simulink model "ammclib_gflib_trigonometric_s32k11x"  (Simulink 9.0)
settings: Solver=FixedStepDiscrete  StartTime=0.0  StopTime=5  FixedStep=0.001  RelTol=1e-3  EnableMultiTasking=on
InitFcn:
  | mbd_s32k_consistency_checks(bdroot(gcs));
undefined symbols (not defined in the file): LQFP, thumb
libraries: ammclib_bam_s32k11x x23, mbd_s32k1xx_ec_toolbox x2, simulink x1
Description:
  | This model tests the AMMCLIB GFLIB TRIGONOMETRIC blocks
  | 
  | Validation:
  | - Run the model in Simulation and check the results
  | - Open Freemaster (ammclib_gflib_trigonometric_s32k11x.pmp) and compare the HW results against the Simulated ones
CloseFcn:
  | clear all;
settings Model: Creator=NXP MBDT Team  LastModifiedBy=nxf35172
settings DataIOCC: ExternalInput=off  InitialState=off  LimitDataPoints=on  SaveOutput=off  SignalLogging=off  SaveTime=off
settings OptimizationCC: DefaultParameterBehavior=Inlined  PassReuseOutputArgsAs=Individual arguments  LifeSpan=auto
settings DebuggingCC: SolverPrmCheckMsg=warning  InheritedTsInSrcMsg=none  SingleTaskRateTransMsg=error  IntegerOverflowMsg=none  ParameterPrecisionLossMsg=none  ParameterTunabilityLossMsg=error  UnconnectedInputMsg=error  UnconnectedOutputMsg=error  UnconnectedLineMsg=error  AllowSymbolicDim=off  UnknownTsInhSupMsg=error  StateNameClashWarn=warning
settings HardwareCC: ProdLargestAtomicInteger=Long  ProdLargestAtomicFloat=Double  ProdIntDivRoundTo=Zero  ProdEndianess=LittleEndian  ProdHWDeviceType=ARM Compatible->ARM Cortex
settings SFSimCC: MATLABDynamicMemAlloc=off
settings RTWCC: SystemTargetFile=mbd_s32k.tlc  MakeCommand=mbd_s32k_make_rtw COPY_MDLREF_INCLUDES=0  TemplateMakefile=mbd_s32k.tmf  Description=Model Based Design Toolbox S32K14x Code Generation Target  GenerateReport=on  IncludeHyperlinkInReport=on  LaunchReport=on  GenerateTraceInfo=on  GenerateTraceReport=on  GenerateTraceReportSl=on  GenerateTraceReportSf=on  GenerateTraceReportEml=on
settings CodeAppCC: ForceParamTrailComments=on  IgnoreCustomStorageClasses=off  OperatorAnnotations=on  SimulinkDataObjDesc=on  SFDataObjDesc=on  InsertBlockDesc=on  StateflowObjectComments=off
settings STFCustomTargetCC: MultiwordLength=256  ModelReferenceCompliant=off  CombineOutputUpdateFcns=on  ERTCustomFileBanners=on  SupportContinuousTime=off  SupportNonInlinedSFcns=off  RemoveResetFunc=on  MATLABClassNameForMDSCustomization=Simulink.SoftwareTarget.ERTCustomization  GRTInterface=off  SystemTargetFile=mbd_s32k.tlc
settings ERTTargetCC: ModelReferenceCompliant=off  ParMdlRefBuildCompliant=off  CompOptLevelCompliant=off  ConcurrentExecutionCompliant=off  ModelStepFunctionPrototypeControlCompliant=off  CPPClassGenCompliant=off  UseToolchainInfoCompliant=off  InlinedParameterPlacement=NonHierarchical  ERTCustomFileTemplate=example_file_process.tlc

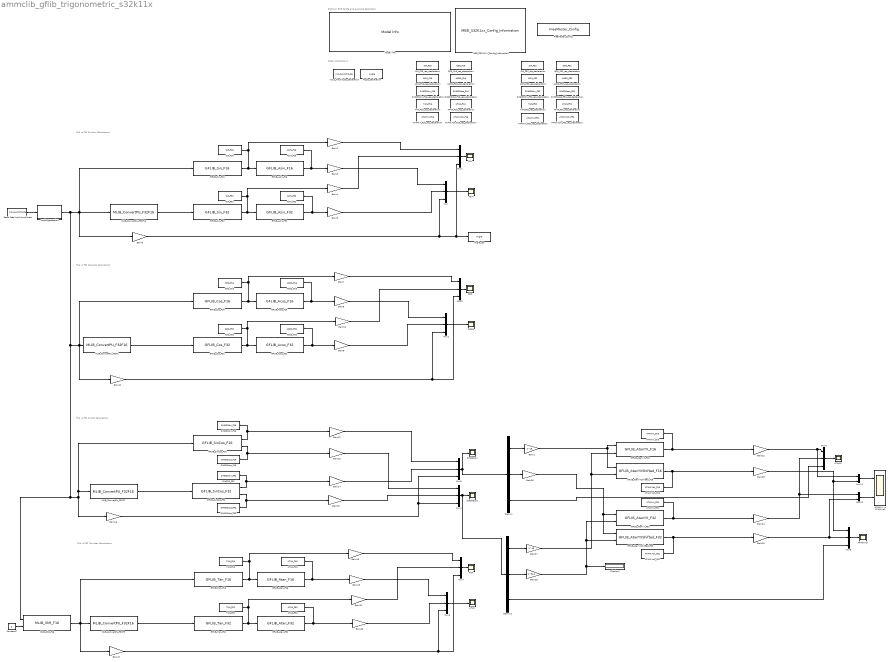
== system ammclib_gflib_trigonometric_s32k11x ==
  note: S32K11x EVB Config and example description
  note: Data Initializations
  note: F16 vs F32 Sin/Asin Calculations
  note: F16 vs F32 Cos/Acos Calculations
  note: F16 vs F32 SinCos Calculations
  note: F16 vs F32 Tan/Atan Calculations
  ACOS : Scope
  ACOS_F16 : DataStoreWrite  DataStoreName=ACOS_F16
  ACOS_F16_res_declaration : DataStoreMemory  Priority=2  DataStoreName=ACOS_F16  ReadBeforeWriteMsg=warning  WriteAfterWriteMsg=warning  WriteAfterReadMsg=warning  ShowAdditionalParam=off  OutDataTypeStr=int16
  ACOS_F32 : DataStoreWrite  DataStoreName=ACOS_F32
  ACOS_F32_res_declaration : DataStoreMemory  Priority=2  DataStoreName=ACOS_F32  ReadBeforeWriteMsg=warning  WriteAfterWriteMsg=warning  WriteAfterReadMsg=warning  ShowAdditionalParam=off  OutDataTypeStr=int32
  ASIN : Scope
  ASIN_F16 : DataStoreWrite  DataStoreName=ASIN_F16
  ASIN_F16_res_declaration : DataStoreMemory  Priority=2  DataStoreName=ASIN_F16  ReadBeforeWriteMsg=warning  WriteAfterWriteMsg=warning  WriteAfterReadMsg=warning  ShowAdditionalParam=off  OutDataTypeStr=int16
  ASIN_F32 : DataStoreWrite  DataStoreName=ASIN_F32
  ASIN_F32_res_declaration : DataStoreMemory  Priority=2  DataStoreName=ASIN_F32  ReadBeforeWriteMsg=warning  WriteAfterWriteMsg=warning  WriteAfterReadMsg=warning  ShowAdditionalParam=off  OutDataTypeStr=int32
  ATAN : Scope
  ATANXY : Scope
  ATANXYsh : Scope
  ATANYX vs ATANXYsh : Scope  NumInputPorts=2
  ATANYX_F16 : DataStoreWrite  DataStoreName=ATANYX_F16
  ATANYX_F16_res_declaration : DataStoreMemory  Priority=2  DataStoreName=ATANYX_F16  ReadBeforeWriteMsg=warning  WriteAfterWriteMsg=warning  WriteAfterReadMsg=warning  ShowAdditionalParam=off  OutDataTypeStr=int16
  ATANYX_F32 : DataStoreWrite  DataStoreName=ATANYX_F32
  ATANYX_F32_res_declaration : DataStoreMemory  Priority=2  DataStoreName=ATANYX_F32  ReadBeforeWriteMsg=warning  WriteAfterWriteMsg=warning  WriteAfterReadMsg=warning  ShowAdditionalParam=off  OutDataTypeStr=int32
  ATANYXsh_F16 : DataStoreWrite  DataStoreName=ATANYXsh_F16
  ATANYXsh_F16_res_declaration : DataStoreMemory  Priority=2  DataStoreName=ATANYXsh_F16  ReadBeforeWriteMsg=warning  WriteAfterWriteMsg=warning  WriteAfterReadMsg=warning  ShowAdditionalParam=off  OutDataTypeStr=int16
  ATANYXsh_F32 : DataStoreWrite  DataStoreName=ATANYXsh_F32
  ATANYXsh_F32_res_declaration : DataStoreMemory  Priority=2  DataStoreName=ATANYXsh_F32  ReadBeforeWriteMsg=warning  WriteAfterWriteMsg=warning  WriteAfterReadMsg=warning  ShowAdditionalParam=off  OutDataTypeStr=int32
  ATAN_F16 : DataStoreWrite  DataStoreName=ATAN_F16
  ATAN_F16_res_declaration : DataStoreMemory  Priority=2  DataStoreName=ATAN_F16  ReadBeforeWriteMsg=warning  WriteAfterWriteMsg=warning  WriteAfterReadMsg=warning  ShowAdditionalParam=off  OutDataTypeStr=int16
  ATAN_F32 : DataStoreWrite  DataStoreName=ATAN_F32
  ATAN_F32_res_declaration : DataStoreMemory  Priority=2  DataStoreName=ATAN_F32  ReadBeforeWriteMsg=warning  WriteAfterWriteMsg=warning  WriteAfterReadMsg=warning  ShowAdditionalParam=off  OutDataTypeStr=int32
  Angle generation : Subsystem
  Angle_declaration : DataStoreMemory  Priority=1  DataStoreName=Angle  WriteAfterWriteMsg=warning  WriteAfterReadMsg=warning  ShowAdditionalParam=off  OutMin=-1  OutMax=1  OutDataTypeStr=single
  Angle_res : DataStoreWrite  DataStoreName=Angle
  COS : Scope
  COS_F16 : DataStoreWrite  DataStoreName=COS_F16
  COS_F16_res_declaration : DataStoreMemory  Priority=2  DataStoreName=COS_F16  ReadBeforeWriteMsg=warning  WriteAfterWriteMsg=warning  WriteAfterReadMsg=warning  ShowAdditionalParam=off  OutDataTypeStr=int16
  COS_F32 : DataStoreWrite  DataStoreName=COS_F32
  COS_F32_res_declaration : DataStoreMemory  Priority=2  DataStoreName=COS_F32  ReadBeforeWriteMsg=warning  WriteAfterWriteMsg=warning  WriteAfterReadMsg=warning  ShowAdditionalParam=off  OutDataTypeStr=int32
  Constant7 : Constant  Value=2  OutDataTypeStr=Inherit: Inherit via back propagation
  Demux : Demux  Outputs=3
  Demux1 : Demux  Outputs=3
  Display2 : Display
  FreeMaster_Config : mbd_s32k1xx_ec_toolbox/Utility Blocks/FreeMaster_Config  interface=LPUART0  baudrate=19200  rxd=PTB0: [LPUART0_RX | Receive]  txd=PTB1: [LPUART0_TX | Transmit]  mode=Short Interrupt  isr_prio=3  show_adv_opts=on  use_scope=on  max_scope_vars=8  use_recorder=on  max_rec_vars=8  rec_buff_size=1024  rec_timebase=0 seconds  comm_buffer_size_auto=on  comm_buffer_size=255  comm_rqueue_size_default=on  comm_rqueue_size=32
  GFLIB_Acos_F16 : ammclib_bam_s32k11x/GFLIB/bam_f16/GFLIB_Acos_F16
  GFLIB_Acos_F32 : ammclib_bam_s32k11x/GFLIB/bam_f32/GFLIB_Acos_F32
  GFLIB_Asin_F16 : ammclib_bam_s32k11x/GFLIB/bam_f16/GFLIB_Asin_F16
  GFLIB_Asin_F32 : ammclib_bam_s32k11x/GFLIB/bam_f32/GFLIB_Asin_F32
  GFLIB_AtanYXShifted_F16 : ammclib_bam_s32k11x/GFLIB/bam_f16/GFLIB_AtanYXShifted_F16  Ky=19918  Kx=28803  Ny=0  Nx=0  ThetaAdj=1820
  GFLIB_AtanYXShifted_F32 : ammclib_bam_s32k11x/GFLIB/bam_f32/GFLIB_AtanYXShifted_F32  Ky=1.305434611595101e+09  Kx=1.887749824036660e+09  Ny=0  Nx=0  ThetaAdj=1.193046470436251e+08
  GFLIB_AtanYX_F16 : ammclib_bam_s32k11x/GFLIB/bam_f16/GFLIB_AtanYX_F16
  GFLIB_AtanYX_F32 : ammclib_bam_s32k11x/GFLIB/bam_f32/GFLIB_AtanYX_F32
  GFLIB_Atan_F16 : ammclib_bam_s32k11x/GFLIB/bam_f16/GFLIB_Atan_F16
  GFLIB_Atan_F32 : ammclib_bam_s32k11x/GFLIB/bam_f32/GFLIB_Atan_F32
  GFLIB_Cos_F16 : ammclib_bam_s32k11x/GFLIB/bam_f16/GFLIB_Cos_F16
  GFLIB_Cos_F32 : ammclib_bam_s32k11x/GFLIB/bam_f32/GFLIB_Cos_F32
  GFLIB_SinCos_F16 : ammclib_bam_s32k11x/GFLIB/bam_f16/GFLIB_SinCos_F16
  GFLIB_SinCos_F32 : ammclib_bam_s32k11x/GFLIB/bam_f32/GFLIB_SinCos_F32
  GFLIB_Sin_F16 : ammclib_bam_s32k11x/GFLIB/bam_f16/GFLIB_Sin_F16
  GFLIB_Sin_F32 : ammclib_bam_s32k11x/GFLIB/bam_f32/GFLIB_Sin_F32
  GFLIB_Tan_F16 : ammclib_bam_s32k11x/GFLIB/bam_f16/GFLIB_Tan_F16
  GFLIB_Tan_F32 : ammclib_bam_s32k11x/GFLIB/bam_f32/GFLIB_Tan_F32
  Gain1 : Gain  Gain=2^15  OutDataTypeStr=int16
  Gain10 : Gain  Gain=1/(2^31)  OutDataTypeStr=single
  Gain{3,6,8,11,16..17,19} (7 alike) : Gain  Gain=pi/(2^15)  OutDataTypeStr=single
  Gain{2,7,12..13,18,22..23} (7 alike) : Gain  Gain=1/(2^15)  OutDataTypeStr=single
  Gain14 : Gain  Gain=1/(2^31-1)  ParamDataTypeStr=double  OutDataTypeStr=single
  Gain15 : Gain  Gain=1/(2^31-1)  ParamDataTypeStr=double  OutDataTypeStr=single
  Gain20 : Gain  Gain=pi/(2^31)  OutDataTypeStr=single
  Gain21 : Gain  Gain=1/(2^31)  OutDataTypeStr=single
  Gain24 : Gain  Gain=1/(2^31)  ParamDataTypeStr=double  OutDataTypeStr=single
  Gain25 : Gain  Gain=1/(2^31-1)  ParamDataTypeStr=double  OutDataTypeStr=single
  Gain26 : Gain  Gain=(2^31-1)  ParamDataTypeStr=double  OutDataTypeStr=int32
  Gain27 : Gain  Gain=2^15  ParamDataTypeStr=int32  OutDataTypeStr=int16
  Gain28 : Gain  Gain=2^31-1  ParamDataTypeStr=double  OutDataTypeStr=int32
  Gain4 : Gain  Gain=1/(2^31)  OutDataTypeStr=single
  Gain5 : Gain  Gain=pi/(2^31)  OutDataTypeStr=single
  Gain9 : Gain  Gain=pi/(2^31)  OutDataTypeStr=single
  Input_Amplitude_declaration : DataStoreMemory  Priority=1  DataStoreName=Input_Amplitude  WriteAfterWriteMsg=warning  WriteAfterReadMsg=warning  InitialValue=3.14  ShowAdditionalParam=off  OutMin=-pi  OutMax=pi  OutDataTypeStr=single
  MBD_S32K11x_Config_Information : mbd_s32k1xx_ec_toolbox/MBD_S32K1xx_Config_Information  mbdt_ver=0  disp_str=|  config_params=[]  mcu_target_name=S32K116  mcu_target_package=48-LQFP  mcu_target_sram_size=17KB  mcu_system_clock_freq=40  mcu_xtal_freq=External 40  mcu_steptick_timer=LPIT Channel 0  mcu_steptick_prio=3  ds_import_enable=on  target_compiler=GCC  target_memory=FLASH  gcc_target_compile_opts=-mcpu=cortex-m0plus -mthumb -O1 -g -gstrict-dwarf  gcc_target_assemble_opts=-mcpu=cortex-m0plus -mthumb -g  gcc_target_link_opts=-mcpu=cortex-m0plus -mthumb  gcc_target_default_lcf=on  gcc_target_user_lcf=S32K116_17_flash.ld  ghs_target_compile_opts=-mcpu=cortexm0plus -mthumb -fsoft -Ogeneral -Wundef -Wimplicit-int -Wshadow -Wtrigraphs --no_commons --gnu_asm -gnu99 -gdwarf-2 -G  ghs_target_assemble_opts=-mcpu=cortexm0plus -mthumb -fsoft --gnu_asm  ghs_target_link_opts=-mcpu=cortexm0plus -mthumb -fsoft  ghs_target_default_lcf=on  ghs_target_user_lcf=S32K116_17_flash.ld  iar_target_compile_opts=--thumb -Ol -e --debug --dlib_config normal  iar_target_assemble_opts=--thumb  iar_target_link_opts=--no_exceptions --vfe --inline  iar_target_default_lcf=on  iar_target_user_lcf=S32K116_17_flash.icf  pil_download_enable=off  rbl_download_enable=on  rbl_start_delay=5000  rbl_download_interface=OpenSDA  rbl_restart_request=off  rbl_com_port=Custom  rbl_com_port_custom=COM1  pil_download_rate=57600  pil_opensda_drive=Custom  pil_opensda_drive_custom=D  pil_uart_instance=0  pil_uart_rx=PTB0: [LPUART0_RX | Receive]  pil_uart_tx=PTB1: [LPUART0_TX | Transmit]  FTM_PWM_PcrCheckEnDis=on  FTM_Input_Edge_Inputs_PcrCheckEnDis=on  FTM_Dual_Edge_Inputs_PcrCheckEnDis=on  FTM_Quadrature_Inputs_PcrCheckEnDis=on  FTM_Hall_Sensor_Inputs_PcrCheckEnDis=on  LPTMR_PcrCheckEnDis=on  PIT_PcrCheckEnDis=on  RTC_PcrCheckEnDis=on  FlexCAN_PcrCheckEnDis=on  LIN_PcrCheckEnDis=on  FlexIO_PcrCheckEnDis=on  LPI2C_PcrCheckEnDis=on  LPSPI_PcrCheckEnDis=on  LPUART_PcrCheckEnDis=on  CMP_PcrCheckEnDis=on  GPIO_OutputPcrCheckEnDis=on  GPIO_InputPcrCheckEnDis=on  SBC_PcrCheckEnDis=on  AMMCLIB_PcrCheckEnDis=on  FM_PcrCheckEnDis=on  Profile_PcrCheckEnDis=on  ConfigParams_PcrCheckEnDis=on  ModelRef_PcrCheckEnDis=on  PDB0_PcrCheckEnDis=on  CSEc_PcrCheckEnDis=on  eDMA_PcrCheckEnDis=on  ADC_PcrCheckEnDis=on  WDOG_PcrCheckEnDis=on
      | Target : S32K144-64KB_SRAM
      | Package : 100-pin
      | System clock : 80 MHz
      | XTAL clock : External 8 MHz
      | Compiler : IAR
      | Target Type : FLASH
      | Download Code after build : off
      | Step Tick Interrupt Priority : 15
  MLIB_ConvertPU_F32F{1..3,16} (4 alike) : ammclib_bam_s32k11x/MLIB/bam_f32/MLIB_ConvertPU_F32F16
  MLIB_ShR_F16 : ammclib_bam_s32k11x/MLIB/bam_f16/MLIB_ShR_F16
  Model Info : simulink/Model-Wide Utilities/Model Info  Frame=off  DisplayStringWithTags=|  HorizontalTextAlignment=Left  LeftAlignmentValue=0.02
      | Model Name: %<ModelName>
      | 
      | Description: %<Description>
  Mux{,1..9} (10 alike) : Mux  Inputs=3
  Mux11 : Mux  Inputs=2
  Mux12 : Mux  Inputs=2
  Read Step Input Amplitude : DataStoreRead  DataStoreName=Input_Amplitude
  SIN : Scope
  SINCOS_F32 : DataStoreWrite  DataStoreName=SINCOSsin_F32
  SINCOScos : Scope
  SINCOScos_F16 : DataStoreWrite  DataStoreName=SINCOScos_F16
  SINCOScos_F16_res_declaration : DataStoreMemory  Priority=2  DataStoreName=SINCOScos_F16  ReadBeforeWriteMsg=warning  WriteAfterWriteMsg=warning  WriteAfterReadMsg=warning  ShowAdditionalParam=off  OutDataTypeStr=int16
  SINCOScos_F32 : DataStoreWrite  DataStoreName=SINCOScos_F32
  SINCOScos_F32_res_declaration : DataStoreMemory  Priority=2  DataStoreName=SINCOScos_F32  ReadBeforeWriteMsg=warning  WriteAfterWriteMsg=warning  WriteAfterReadMsg=warning  ShowAdditionalParam=off  OutDataTypeStr=int32
  SINCOSsin : Scope
  SINCOSsin_F16 : DataStoreWrite  DataStoreName=SINCOSsin_F16
  SINCOSsin_F16_res_declaration : DataStoreMemory  Priority=2  DataStoreName=SINCOSsin_F16  ReadBeforeWriteMsg=warning  WriteAfterWriteMsg=warning  WriteAfterReadMsg=warning  ShowAdditionalParam=off  OutDataTypeStr=int16
  SINCOSsin_F32_res_declaration : DataStoreMemory  Priority=2  DataStoreName=SINCOSsin_F32  ReadBeforeWriteMsg=warning  WriteAfterWriteMsg=warning  WriteAfterReadMsg=warning  ShowAdditionalParam=off  OutDataTypeStr=int32
  SIN_F16 : DataStoreWrite  DataStoreName=SIN_F16
  SIN_F16_res_declaration : DataStoreMemory  Priority=2  DataStoreName=SIN_F16  ReadBeforeWriteMsg=warning  WriteAfterWriteMsg=warning  WriteAfterReadMsg=warning  ShowAdditionalParam=off  OutDataTypeStr=int16
  SIN_F32 : DataStoreWrite  DataStoreName=SIN_F32
  SIN_F32_res_declaration : DataStoreMemory  Priority=2  DataStoreName=SIN_F32  ReadBeforeWriteMsg=warning  WriteAfterWriteMsg=warning  WriteAfterReadMsg=warning  ShowAdditionalParam=off  OutDataTypeStr=int32
  TAN : Scope
  TAN_F16 : DataStoreWrite  DataStoreName=TAN_F16
  TAN_F16_res_declaration : DataStoreMemory  Priority=2  DataStoreName=TAN_F16  ReadBeforeWriteMsg=warning  WriteAfterWriteMsg=warning  WriteAfterReadMsg=warning  ShowAdditionalParam=off  OutDataTypeStr=int16
  TAN_F32 : DataStoreWrite  DataStoreName=TAN_F32
  TAN_F32_res_declaration : DataStoreMemory  Priority=2  DataStoreName=TAN_F32  ReadBeforeWriteMsg=warning  WriteAfterWriteMsg=warning  WriteAfterReadMsg=warning  ShowAdditionalParam=off  OutDataTypeStr=int32
  wires:
  MLIB_ConvertPU_F32F16/1 -> GFLIB_Sin_F32/1
  GFLIB_Sin_F32/1 -> Gain4/1, SIN_F32/1, GFLIB_Asin_F32/1
  Gain6/1 -> Mux/3, Mux1/3, Angle_res/1  "Angle[rad]"
  Mux/1 -> ASIN/1
  GFLIB_Asin_F16/1 -> Gain3/1, ASIN_F16/1
  GFLIB_Asin_F32/1 -> Gain5/1, ASIN_F32/1
  Gain3/1 -> Mux/1  "ASIN_F16"
  Gain5/1 -> Mux/2  "ASIN_F32"
  Mux1/1 -> SIN/1
  Gain2/1 -> Mux1/1  "SIN_F16"
  Gain4/1 -> Mux1/2  "SIN_F32"
  Read Step Input Amplitude/1 -> Angle generation/1("Amplitude ")
  GFLIB_Cos_F16/1 -> GFLIB_Acos_F16/1, Gain7/1, COS_F16/1
  MLIB_ConvertPU_F32F1/1 -> GFLIB_Cos_F32/1
  GFLIB_Cos_F32/1 -> GFLIB_Acos_F32/1, Gain10/1, COS_F32/1
  Gain11/1 -> Mux2/3, Mux3/3  "Angle[rad]"
  Mux2/1 -> ACOS/1
  GFLIB_Acos_F16/1 -> Gain8/1, ACOS_F16/1
  GFLIB_Acos_F32/1 -> Gain9/1, ACOS_F32/1
  Gain8/1 -> Mux2/1  "ACOS_F16"
  Gain9/1 -> Mux2/2  "ACOS_F32"
  Mux3/1 -> COS/1
  Gain7/1 -> Mux3/1  "COS_F16"
  Gain10/1 -> Mux3/2  "COS_F32"
  GFLIB_SinCos_F16/1 -> Gain12/1, SINCOSsin_F16/1
  MLIB_ConvertPU_F32F2/1 -> GFLIB_SinCos_F32/1
  GFLIB_SinCos_F32/1 -> Gain14/1, SINCOS_F32/1
  Mux5/1 -> SINCOSsin/1, Demux/1
  Gain12/1 -> Mux5/1  "SINCOSsin_F16"
  Gain14/1 -> Mux5/2  "SINCOSsin_F32"
  GFLIB_SinCos_F16/2 -> Gain13/1, SINCOScos_F16/1
  GFLIB_SinCos_F32/2 -> Gain15/1, SINCOScos_F32/1
  Mux4/1 -> Demux1/1, SINCOScos/1
  Gain13/1 -> Mux4/1  "SINCOScos_F16"
  Gain15/1 -> Mux4/2  "SINCOScos-F32"
  GFLIB_Tan_F16/1 -> GFLIB_Atan_F16/1, Gain18/1, TAN_F16/1
  MLIB_ConvertPU_F32F3/1 -> GFLIB_Tan_F32/1
  GFLIB_Tan_F32/1 -> GFLIB_Atan_F32/1, Gain21/1, TAN_F32/1
  Gain17/1 -> Mux7/3, Mux6/3  "Angle[rad]"
  Mux6/1 -> ATAN/1
  GFLIB_Atan_F16/1 -> Gain19/1, ATAN_F16/1
  GFLIB_Atan_F32/1 -> Gain20/1, ATAN_F32/1
  Gain19/1 -> Mux6/1  "ATAN_F16"
  Gain20/1 -> Mux6/2  "ATAN_F32"
  Mux7/1 -> TAN/1
  Gain18/1 -> Mux7/1  "TAN_F16"
  Gain21/1 -> Mux7/2  "TAN_F32"
  Constant7/1 -> MLIB_ShR_F16/2
  GFLIB_AtanYX_F16/1 -> Gain22/1, ATANYX_F16/1
  GFLIB_AtanYX_F32/1 -> Gain24/1, ATANYX_F32/1
  Gain16/1 -> Mux4/3, Mux5/3  "Angle[rad]"
  Mux8/1 -> ATANXYsh/1
  GFLIB_AtanYXShifted_F16/1 -> Gain23/1, ATANYXsh_F16/1
  Gain23/1 -> Mux11/2, Mux8/1  "ATANsh_F16"
  Gain25/1 -> Mux12/2, Mux8/2  "ATANsh_F32"
  Mux9/1 -> ATANXY/1
  Gain22/1 -> Mux11/1, Mux9/1  "ATANYX_F16"
  Gain24/1 -> Mux9/2, Mux12/1  "ATANYX_F32"
  Angle generation/1(Angle) -> MLIB_ShR_F16/1, MLIB_ConvertPU_F32F2/1, GFLIB_SinCos_F16/1, Gain16/1, Gain11/1, GFLIB_Cos_F16/1, MLIB_ConvertPU_F32F1/1, Gain6/1, GFLIB_Sin_F16/1, MLIB_ConvertPU_F32F16/1
  GFLIB_AtanYXShifted_F32/1 -> Gain25/1, ATANYXsh_F32/1
  Demux/1 -> Gain1/1
  Demux1/1 -> Gain27/1
  Demux1/2 -> Gain28/1
  Demux1/3 -> Mux8/3
  Gain1/1 -> GFLIB_AtanYX_F16/1, GFLIB_AtanYXShifted_F16/1
  Gain26/1 -> GFLIB_AtanYX_F32/1, GFLIB_AtanYXShifted_F32/1
  Gain27/1 -> GFLIB_AtanYXShifted_F16/2, GFLIB_AtanYX_F16/2
  Gain28/1 -> Display2/1, GFLIB_AtanYX_F32/2, GFLIB_AtanYXShifted_F32/2
  GFLIB_Sin_F16/1 -> Gain2/1, SIN_F16/1, GFLIB_Asin_F16/1
  MLIB_ShR_F16/1 -> GFLIB_Tan_F16/1, Gain17/1, MLIB_ConvertPU_F32F3/1
  Demux/3 -> Mux9/3
  Mux11/1 -> ATANYX vs ATANXYsh/1
  Mux12/1 -> ATANYX vs ATANXYsh/2
  Demux/2 -> Gain26/1

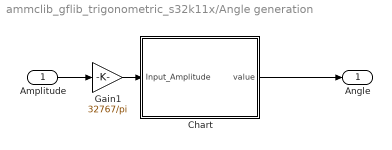
== system ammclib_gflib_trigonometric_s32k11x/Angle generation ==
  "Amplitude " : Inport
  Chart : Stateflow chart  TreatAsAtomicUnit=on
  Gain1 : Gain  Gain=32767/pi  OutDataTypeStr=Inherit: Inherit via back propagation
  Angle : Outport
  wires:
  Chart/1(value) -> Angle/1
  "Amplitude "/1 -> Gain1/1
  Gain1/1 -> Chart/1(Input_Amplitude)

== stateflow chart Angle generation/Chart ==
  settings: executeAtInitialization=1
  state A
    du:
    cntr=cntr+25;
    value=cntr;
    ex:
    cntr = -Input_Amplitude;
  (default) -> A : {cntr=0;}
  A -> A : [cntr >= Input_Amplitude]
  data: cntr local int16 =0; value output int16; Input_Amplitude input int16
